simulink model "Pendulosimple_Linealizacions"  (R2017b)
settings: Solver=ode5  StartTime=0.0  StopTime=10  FixedStep=0.0001  RelTol=1e-3
values from neighbouring files (symbols this model uses):
  Api = [0 1 ... (first row only)    [Pendulosimple_Linealizacion.m]
  B = [0;1/I]    [Pendulosimple_Linealizacion.m]    (also in furuta.m = [0;-2740.545688;0;2772.787402])
  beta = 0.0005    [Pendulosimple_Linealizacion.m]
  C = [1 0]    [Pendulosimple_Linealizacion.m]    (also in furuta.m = [0 0 1 0])
  g = 9.81    [Pendulosimple_Linealizacion.m]
  I = 1*m*L^2/12    (= 3.3282e-05)    [Pendulosimple_Linealizacion.m]
  K = place(Api,B,p)    [Pendulosimple_Linealizacion.m]
  Lpcm = L/2    (= 0.0645)    [Pendulosimple_Linealizacion.m]    (also in furuta.m)
  m = 0.024    [Pendulosimple_Linealizacion.m]
libraries: aerolibconvert2 x2
settings Model: Creator=luism  LastModifiedBy=luism

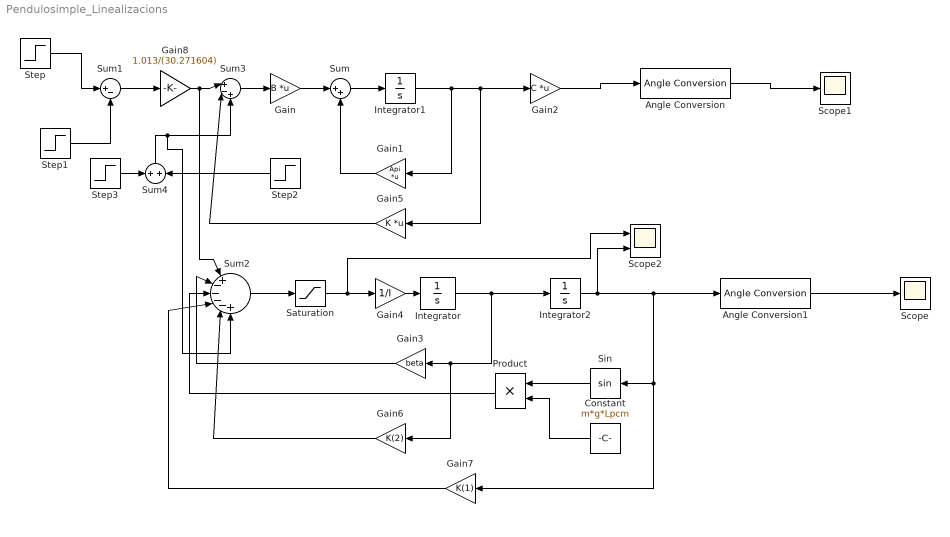
== system Pendulosimple_Linealizacions ==
  Angle Conversion : aerolibconvert2/Angle Conversion  IU=rad  OU=deg
  Angle Conversion1 : aerolibconvert2/Angle Conversion  IU=rad  OU=deg
  Constant : Constant  Value=m*g*Lpcm
  Gain : Gain  Gain=B  Multiplication=Matrix(K*u)
  Gain1 : Gain  Gain=Api  Multiplication=Matrix(K*u)
  Gain2 : Gain  Gain=C  Multiplication=Matrix(K*u)
  Gain3 : Gain  Gain=beta
  Gain4 : Gain  Gain=1/I
  Gain5 : Gain  Gain=K  Multiplication=Matrix(K*u)
  Gain6 : Gain  Gain=K(2)
  Gain7 : Gain  Gain=K(1)
  Gain8 : Gain  Gain=1.013/(30.271604)
  Integrator : Integrator
  Integrator1 : Integrator  InitialCondition=[0,0]
  Integrator2 : Integrator  InitialCondition=pi
  Product : Product
  Saturation : Saturate  UpperLimit=0.1  LowerLimit=-0.1
  Scope : Scope
  Scope1 : Scope
  Scope2 : Scope  NumInputPorts=2
  Sin : Trigonometry
  Step : Step  Time=0  After=pi  SampleTime=0
  Step1 : Step  Time=0.2  After=0  SampleTime=0
  Step2 : Step  Time=1.2  After=-2  SampleTime=0
  Step3 : Step  After=2  SampleTime=0
  Sum : Sum  Inputs=|++
  Sum1 : Sum  Inputs=|+-
  Sum2 : Sum  Inputs=|+----+
  Sum3 : Sum  Inputs=|+-+
  Sum4 : Sum  Inputs=+|+
  wires:
  Sum/1 -> Integrator1/1
  Gain1/1 -> Sum/2
  Integrator1/1 -> Gain5/1, Gain2/1, Gain1/1
  Gain/1 -> Sum/1
  Step1/1 -> Sum1/2
  Step/1 -> Sum1/1
  Integrator/1 -> Gain6/1, Gain3/1, Integrator2/1
  Gain3/1 -> Sum2/2
  Sin/1 -> Product/1
  Constant/1 -> Product/2
  Product/1 -> Sum2/3
  Gain5/1 -> Sum3/2
  Sum3/1 -> Gain/1
  Gain8/1 -> Sum2/1, Sum3/1
  Sum1/1 -> Gain8/1
  Gain4/1 -> Integrator/1
  Gain6/1 -> Sum2/5
  Gain7/1 -> Sum2/4
  Gain2/1 -> Angle Conversion/1
  Angle Conversion/1 -> Scope1/1
  Angle Conversion1/1 -> Scope/1
  Step3/1 -> Sum4/1
  Step2/1 -> Sum4/2
  Sum4/1 -> Sum2/6, Sum3/3
  Integrator2/1 -> Scope2/2, Angle Conversion1/1, Sin/1, Gain7/1
  Sum2/1 -> Saturation/1
  Saturation/1 -> Scope2/1, Gain4/1
